simulink model "right_leg"  (R2014b)
settings: Solver=ode45  StartTime=0.0  StopTime=10  FixedStep=1e-3  RelTol=1e-3
undefined symbols (not defined in the file or in its folder): MX28_inertia, MX28_init_position, MX28_init_speed, MX28_Te, X, Y, Z
libraries: sm_lib x39, nesl_utility x20
(part 1 of 2)
settings Model: Creator=florent  LastModifiedBy=florent
settings DebuggingCC: IntegerOverflowMsg=none  ParameterDowncastMsg=warning  ParameterPrecisionLossMsg=none  ParameterTunabilityLossMsg=none  StateNameClashWarn=warning  IntegerSaturationMsg=none
settings DiagnosticsConfigSet: SimMechanicsConflictingReferenceFrames=none

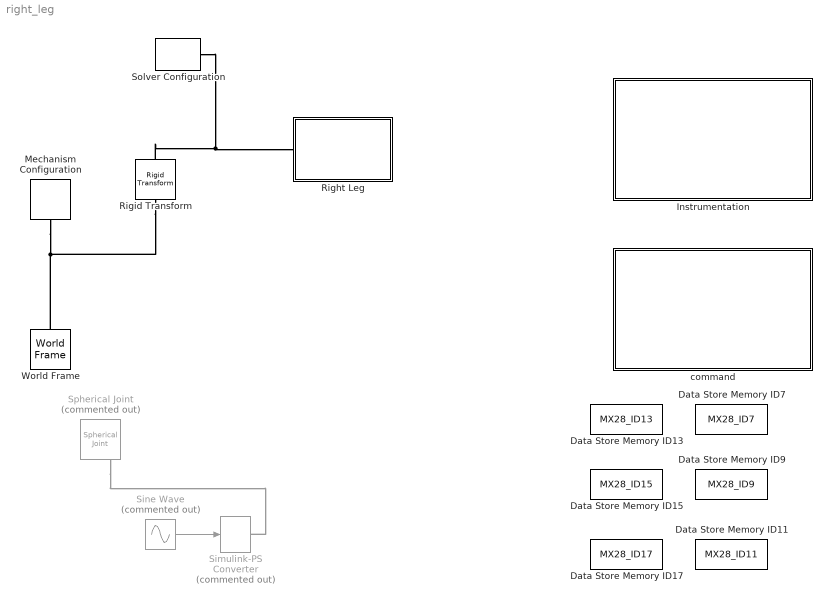
== system right_leg ==
  Data Store Memory ID11 : DataStoreMemory  DataStoreName=MX28_ID11  WriteAfterWriteMsg=error  InitialValue=MX28_default  VectorParams1D=off  OutDataTypeStr=Bus: MX28_bus
  Data Store Memory ID13 : DataStoreMemory  DataStoreName=MX28_ID13  WriteAfterWriteMsg=error  InitialValue=MX28_default  VectorParams1D=off  OutDataTypeStr=Bus: MX28_bus
  Data Store Memory ID15 : DataStoreMemory  DataStoreName=MX28_ID15  WriteAfterWriteMsg=error  InitialValue=MX28_default  VectorParams1D=off  OutDataTypeStr=Bus: MX28_bus
  Data Store Memory ID17 : DataStoreMemory  DataStoreName=MX28_ID17  WriteAfterWriteMsg=error  InitialValue=MX28_default  VectorParams1D=off  OutDataTypeStr=Bus: MX28_bus
  Data Store Memory ID7 : DataStoreMemory  DataStoreName=MX28_ID7  WriteAfterWriteMsg=error  InitialValue=MX28_default  VectorParams1D=off  OutDataTypeStr=Bus: MX28_bus
  Data Store Memory ID9 : DataStoreMemory  DataStoreName=MX28_ID9  WriteAfterWriteMsg=error  InitialValue=MX28_default  VectorParams1D=off  OutDataTypeStr=Bus: MX28_bus
  Instrumentation : Subsystem
  Mechanism Configuration : sm_lib/Utilities/Mechanism Configuration  UniformGravity=Constant  GravityVector=[0 0 -9.80665]  GravityUnits=m/s^2  LinearizationDelta=0.0001  BlockFunction=simmechanics.library.utilities.mechanism_configuration
  Right Leg : Subsystem
      mask init:
      | [ModelDir,~,~] = fileparts(which(gcs));
      | 
      | Block = [gcb '/Right Hip Yaw/Solid'];
      | STLFileName = [ModelDir filesep 'STL' filesep 'Hip1.STL'];
      | if ~strcmp(get_param(Block,'ExtGeomFileName'),STLFileName)
      |     set_param(Block,'ExtGeomFileName',STLFileName);
      | end
      | 
      | Block = [gcb '/Right Hip Roll/Solid'];
      | STLFileName = [ModelDir filesep 'STL' filesep 'Right_Hip2.STL'];
      | if ~strcmp(get_param(Block,'ExtGeomFileName'),STLFileName)
      |     set_param(Block,'ExtGeomFileName',STLFileName);
      | end
      | 
      | Block = [gcb '/Right Thigh/Solid'];
      | STLFileName = [ModelDir filesep 'STL' filesep 'Right_Thigh.STL'];
      | if ~strcmp(get_param(Block,'ExtGeomFileName'),STLFileName)
      |     set_param(Block,'ExtGeomFileName',STLFileName);
      | end
      | 
      | Block = [gcb '/Right Lower Leg/Solid'];
      | STLFileName = [ModelDir filesep 'STL' filesep 'Right_Lower_Leg.STL'];
      | if ~strcmp(get_param(Block,'ExtGeomFileName'),STLFileName)
      |     set_param(Block,'ExtGeomFileName',STLFileName);
      | end
      | 
      | Block = [gcb '/Right Ankle/Solid'];
      | STLFileName = [ModelDir filesep 'STL' filesep 'Right_Ankle.STL'];
      | if ~strcmp(get_param(Block,'ExtGeomFileName'),STLFileName)
      |     set_param(Block,'ExtGeomFileName',STLFileName);
      | end
      | 
      | Block = [gcb '/Right Foot/Solid'];
      | STLFileName = [ModelDir filesep 'STL' filesep 'Right_Foot.STL'];
      | if ~strcmp(get_param(Block,'ExtGeomFileName'),STLFileName)
      |     set_param(Block,'ExtGeomFileName',STLFileName);
      | end
  Rigid Transform : sm_lib/Frames and Transforms/Rigid Transform  TranslationMethod=Cartesian  TranslationLengthUnit=m  TranslationStandardAxis=+Z  TranslationStandardOffset=0  TranslationCartesianOffset=[0 -0.001 0]  TranslationROffset=0  TranslationROffsetUnits=m  TranslationZOffset=0  TranslationZOffsetUnits=m  TranslationThetaOffset=0  TranslationThetaOffsetUnits=deg  RotationMethod=AlignedAxes  RotationAngleUnits=deg  RotationStandardAxis=+Z  RotationAngle=0  RotationArbitraryAxis=[0 0 1]  FollAlignAxisA=+Z  BaseAlignAxisA=-Z  FollAlignAxisB=+X  BaseAlignAxisB=-Y  RotationMatrix=[1 0 0; 0 1 0; 0 0 1]  BlockFunction=simmechanics.library.frames_transforms.rigid_transform
  Simulink-PS Converter : nesl_utility/Simulink-PS Converter  Commented=on  PhysicalDomain=network_engine_domain  SubClassName=ps_input  LeftPortType=input  RightPortType=output  PseudoPeriodic=off  Frequencies=[]  NoiseDistribution=none  NoiseParameters=[]  Unit=1  AffineConversion=off  InputFiltering=off  SimscapeFilterOrder=1  InputFilterTimeConstant=0.001  UdotUserProvided=1
  Sine Wave : Sin  Commented=on  Amplitude=0.1  Frequency=10  SampleTime=0
  Solver Configuration : nesl_utility/Solver Configuration  PhysicalDomain=network_engine_domain  SubClassName=solver  LeftPortType=input  RightPortType=generic  Accelerate=off  Tones=[]  Harmonics=[]  SimulateNoise=off  Profile=off  UseLocalSampling=off  EnableSwitchedLinearOptims=on  FrequencyDomain=off  UseCCode=off  RelTol=0.001  AbsTol=1e-06  MinStep=1e-09  ToWorkspace=off  DoDC=off  ResidualTolerance=1e-05  UseLocalSolver=off  LocalSolverChoice=NE_BACKWARD_EULER_ADVANCER  LocalSolverSampleTime=0.001  DoFixedCost=off  MaxNonlinIter=3  MaxModeIter=2  LinearAlgebra=Sparse  DelaysMemoryBudget=1024  AutomaticFiltering=on  FilteringTimeConstant=0.001
  Spherical Joint : sm_lib/Joints/Spherical Joint  Commented=on  SenseConstraintForce=off  SenseConstraintForceX=off  SenseConstraintForceY=off  SenseConstraintForceZ=off  SenseConstraintTorque=off  SenseConstraintTorqueX=off  SenseConstraintTorqueY=off  SenseConstraintTorqueZ=off  SenseTotalForce=off  SenseTotalForceX=off  SenseTotalForceY=off  SenseTotalForceZ=off  SenseTotalTorque=off  SenseTotalTorqueX=off  SenseTotalTorqueY=off  SenseTotalTorqueZ=off  CompositeWrenchDir=FollowerOnBase  CompositeWrenchFrame=BaseFrame  DefPosRotationMethod=None  DefPosRotationAngleUnits=deg  DefPosRotationStandardAxis=+Z  DefPosRotationAngle=0  DefPosRotationArbitraryAxis=[0 0 1]  DefPosFollAlignAxisA=+X  DefPosBaseAlignAxisA=+Y  DefPosFollAlignAxisB=+Y  DefPosBaseAlignAxisB=+Z  DefPosRotationMatrix=[1 0 0; 0 1 0; 0 0 1]  EqPosRotationMethod=None  EqPosRotationAngleUnits=deg  EqPosRotationStandardAxis=+Z  EqPosRotationAngle=0  EqPosRotationArbitraryAxis=[0 0 1]  EqPosFollAlignAxisA=+X  EqPosBaseAlignAxisA=+Y  EqPosFollAlignAxisB=+Y  EqPosBaseAlignAxisB=+Z  EqPosRotationMatrix=[1 0 0; 0 1 0; 0 0 1]  SpringStiffness=0  SpringStiffnessUnits=N*m/deg  DampingCoefficient=0  DampingCoefficientUnits=N*m/(deg/s)  ActuateTorqueX=off  ActuateTorqueY=on  ActuateTorqueZ=off  ActuateTorque=off  TorqueActuationMode=InputTorque  MotionActuationMode=ComputedMotion  ActuationFrame=BaseFrame  SensePosition=off  SenseVelocityX=off  SenseVelocityY=off  SenseVelocityZ=off  SenseVelocity=off  SenseAccelerationX=off  SenseAccelerationY=off  SenseAccelerationZ=off  SenseAcceleration=off  SenseTorqueX=off  SenseTorqueY=off  SenseTorqueZ=off  SenseTorqueForce=off  SensingFrame=BaseFrame  PositionTargetRotationMethod=ArbitraryAxis  PositionTargetRotationAngleUnits=deg  PositionTargetRotationStandardAxis=+Z  PositionTargetRotationAngle=0  PositionTargetRotationArbitraryAxis=[0 -1 0]  PositionTargetFollAlignAxisA=+X  PositionTargetBaseAlignAxisA=+Y  PositionTargetFollAlignAxisB=+Y  PositionTargetBaseAlignAxisB=+Z  PositionTargetRotationMatrix=[1 0 0; 0 1 0; 0 0 1]  PositionTargetSpecify=on  PositionTargetPriority=High  VelocityTargetValue=[0 0 0]  VelocityTargetValueUnits=deg/s  VelocityTargetSpecify=off  VelocityTargetPriority=High  VelocityTargetInFollowerFrame=on  BlockFunction=simmechanics.library.joints.spherical_joint
  World Frame : sm_lib/Frames and Transforms/World Frame  BlockFunction=simmechanics.library.frames_transforms.world_frame
  command : Subsystem
  wires:
  Sine Wave/1 -> Simulink-PS Converter/1
  connections:
  Solver Configuration/RConn1 -- Rigid Transform/RConn1 -- Right Leg/LConn1
  World Frame/RConn1 -- Rigid Transform/LConn1 -- Mechanism Configuration/RConn1
  Spherical Joint/LConn2 -- Simulink-PS Converter/RConn1

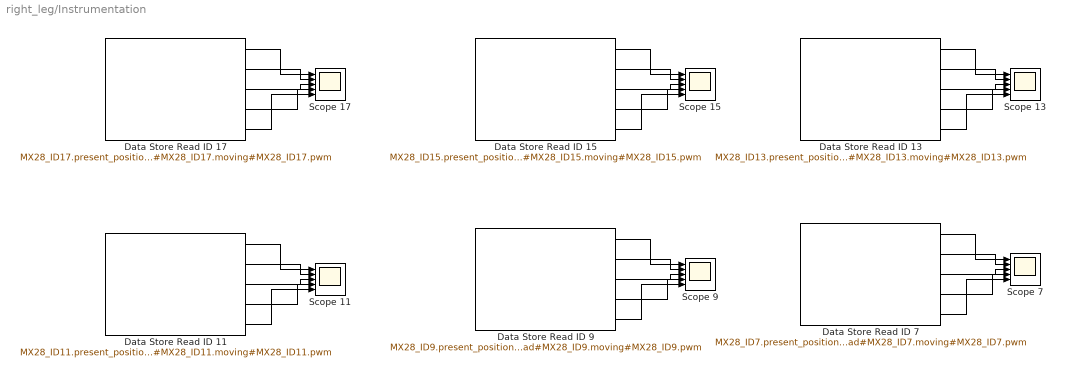
== system right_leg/Instrumentation ==
  Data Store Read ID 11 : DataStoreRead  DataStoreName=MX28_ID11  SampleTime=0.001  DataStoreElements=MX28_ID11.present_position#MX28_ID11.present_speed#MX28_ID11.present_load#MX28_ID11.moving#MX28_ID11.pwm
  Data Store Read ID 13 : DataStoreRead  DataStoreName=MX28_ID13  SampleTime=0.001  DataStoreElements=MX28_ID13.present_position#MX28_ID13.present_speed#MX28_ID13.present_load#MX28_ID13.moving#MX28_ID13.pwm
  Data Store Read ID 15 : DataStoreRead  DataStoreName=MX28_ID15  SampleTime=0.001  DataStoreElements=MX28_ID15.present_position#MX28_ID15.present_speed#MX28_ID15.present_load#MX28_ID15.moving#MX28_ID15.pwm
  Data Store Read ID 17 : DataStoreRead  DataStoreName=MX28_ID17  SampleTime=0.001  DataStoreElements=MX28_ID17.present_position#MX28_ID17.present_speed#MX28_ID17.present_load#MX28_ID17.moving#MX28_ID17.pwm
  Data Store Read ID 7 : DataStoreRead  DataStoreName=MX28_ID7  SampleTime=0.001  DataStoreElements=MX28_ID7.present_position#MX28_ID7.present_speed#MX28_ID7.present_load#MX28_ID7.moving#MX28_ID7.pwm
  Data Store Read ID 9 : DataStoreRead  DataStoreName=MX28_ID9  SampleTime=0.001  DataStoreElements=MX28_ID9.present_position#MX28_ID9.present_speed#MX28_ID9.present_load#MX28_ID9.moving#MX28_ID9.pwm
  Scope {7,9,11,13,15,17} (6 alike) : Scope  NumInputPorts=5
      Scope 11 settings: YMin=-5~0~-5~-5~-5  YMax=5~650~5~5~5
      Scope 13 settings: YMin=2046~-5~-40~-1~0  YMax=2047~5~0~1~20
      Scope 15 settings: YMin=2049~-5~0~-1~-20  YMax=2050~5~40~1~0  SaveName=ScopeData3
      Scope 17 settings: YMin=2048~-5~-20~-1~-10  YMax=2049~5~20~1~0  SaveName=ScopeData4
      Scope 7 settings: YMin=-5~0~-5~-5~-5  YMax=5~650~5~5~5  SaveName=ScopeData6
      Scope 9 settings: YMin=-5~0~-5~-5~-5  YMax=5~650~5~5~5  SaveName=ScopeData5
  wires:
  Data Store Read ID 13/1 -> Scope 13/1
  Data Store Read ID 13/2 -> Scope 13/2
  Data Store Read ID 13/3 -> Scope 13/3
  Data Store Read ID 13/4 -> Scope 13/4
  Data Store Read ID 13/5 -> Scope 13/5
  Data Store Read ID 15/1 -> Scope 15/1
  Data Store Read ID 15/2 -> Scope 15/2
  Data Store Read ID 15/3 -> Scope 15/3
  Data Store Read ID 15/4 -> Scope 15/4
  Data Store Read ID 15/5 -> Scope 15/5
  Data Store Read ID 17/1 -> Scope 17/1
  Data Store Read ID 17/2 -> Scope 17/2
  Data Store Read ID 17/3 -> Scope 17/3
  Data Store Read ID 17/4 -> Scope 17/4
  Data Store Read ID 17/5 -> Scope 17/5
  Data Store Read ID 11/1 -> Scope 11/1
  Data Store Read ID 11/2 -> Scope 11/2
  Data Store Read ID 11/3 -> Scope 11/3
  Data Store Read ID 11/4 -> Scope 11/4
  Data Store Read ID 11/5 -> Scope 11/5
  Data Store Read ID 9/1 -> Scope 9/1
  Data Store Read ID 9/2 -> Scope 9/2
  Data Store Read ID 9/3 -> Scope 9/3
  Data Store Read ID 9/4 -> Scope 9/4
  Data Store Read ID 9/5 -> Scope 9/5
  Data Store Read ID 7/1 -> Scope 7/1
  Data Store Read ID 7/2 -> Scope 7/2
  Data Store Read ID 7/3 -> Scope 7/3
  Data Store Read ID 7/4 -> Scope 7/4
  Data Store Read ID 7/5 -> Scope 7/5

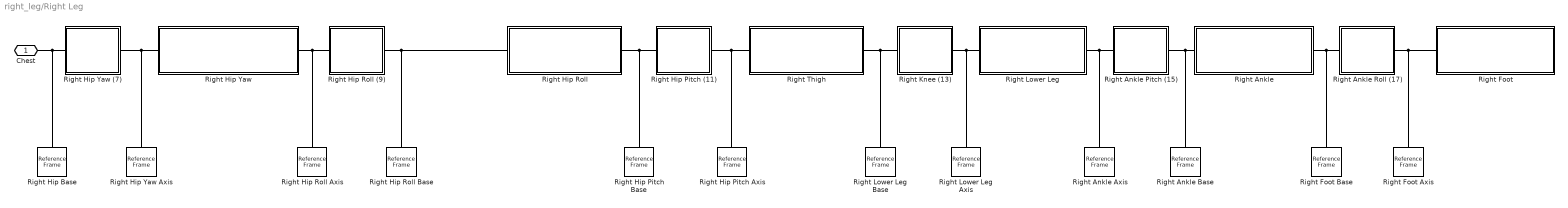
== system right_leg/Right Leg ==
  Right Ankle : Subsystem
  Right Ankle Axis : sm_lib/Frames and Transforms/Reference Frame  BlockFunction=simmechanics.library.frames_transforms.reference_frame
  Right Ankle Base : sm_lib/Frames and Transforms/Reference Frame  BlockFunction=simmechanics.library.frames_transforms.reference_frame
  Right Ankle Pitch (15) : Subsystem
  Right Ankle Roll (17) : Subsystem
  Right Foot : Subsystem
  Right Foot Axis : sm_lib/Frames and Transforms/Reference Frame  BlockFunction=simmechanics.library.frames_transforms.reference_frame
  Right Foot Base : sm_lib/Frames and Transforms/Reference Frame  BlockFunction=simmechanics.library.frames_transforms.reference_frame
  Right Hip Base : sm_lib/Frames and Transforms/Reference Frame  BlockFunction=simmechanics.library.frames_transforms.reference_frame
  Right Hip Pitch (11) : Subsystem
  Right Hip Pitch Axis : sm_lib/Frames and Transforms/Reference Frame  BlockFunction=simmechanics.library.frames_transforms.reference_frame
  Right Hip Pitch Base : sm_lib/Frames and Transforms/Reference Frame  BlockFunction=simmechanics.library.frames_transforms.reference_frame
  Right Hip Roll : Subsystem
  Right Hip Roll (9) : Subsystem
  Right Hip Roll Axis : sm_lib/Frames and Transforms/Reference Frame  BlockFunction=simmechanics.library.frames_transforms.reference_frame
  Right Hip Roll Base : sm_lib/Frames and Transforms/Reference Frame  BlockFunction=simmechanics.library.frames_transforms.reference_frame
  Right Hip Yaw : Subsystem
  Right Hip Yaw (7) : Subsystem
  Right Hip Yaw Axis : sm_lib/Frames and Transforms/Reference Frame  BlockFunction=simmechanics.library.frames_transforms.reference_frame
  Right Knee (13) : Subsystem
  Right Lower Leg : Subsystem
  Right Lower Leg Axis : sm_lib/Frames and Transforms/Reference Frame  BlockFunction=simmechanics.library.frames_transforms.reference_frame
  Right Lower Leg Base : sm_lib/Frames and Transforms/Reference Frame  BlockFunction=simmechanics.library.frames_transforms.reference_frame
  Right Thigh : Subsystem
  Chest : PMIOPort  Port=1  Side=Left
  connections:
  Chest/RConn1 -- Right Hip Yaw (7)/LConn1 -- Right Hip Base/RConn1
  Right Hip Yaw Axis/RConn1 -- Right Hip Yaw (7)/RConn1 -- Right Hip Yaw/LConn1
  Right Hip Yaw/RConn1 -- Right Hip Roll (9)/RConn1 -- Right Hip Roll Axis/RConn1
  Right Hip Roll/RConn1 -- Right Hip Pitch Base/RConn1 -- Right Hip Pitch (11)/LConn1
  Right Thigh/RConn1 -- Right Lower Leg Base/RConn1 -- Right Knee (13)/LConn1
  Right Ankle/RConn1 -- Right Foot Base/RConn1 -- Right Ankle Roll (17)/LConn1
  Right Thigh/LConn1 -- Right Hip Pitch (11)/RConn1 -- Right Hip Pitch Axis/RConn1
  Right Lower Leg/LConn1 -- Right Knee (13)/RConn1 -- Right Lower Leg Axis/RConn1
  Right Lower Leg/RConn1 -- Right Ankle Axis/RConn1 -- Right Ankle Pitch (15)/RConn1
  Right Ankle/LConn1 -- Right Ankle Pitch (15)/LConn1 -- Right Ankle Base/RConn1
  Right Ankle Roll (17)/RConn1 -- Right Foot/LConn1 -- Right Foot Axis/RConn1
  Right Hip Roll Base/RConn1 -- Right Hip Roll (9)/LConn1 -- Right Hip Roll/LConn1

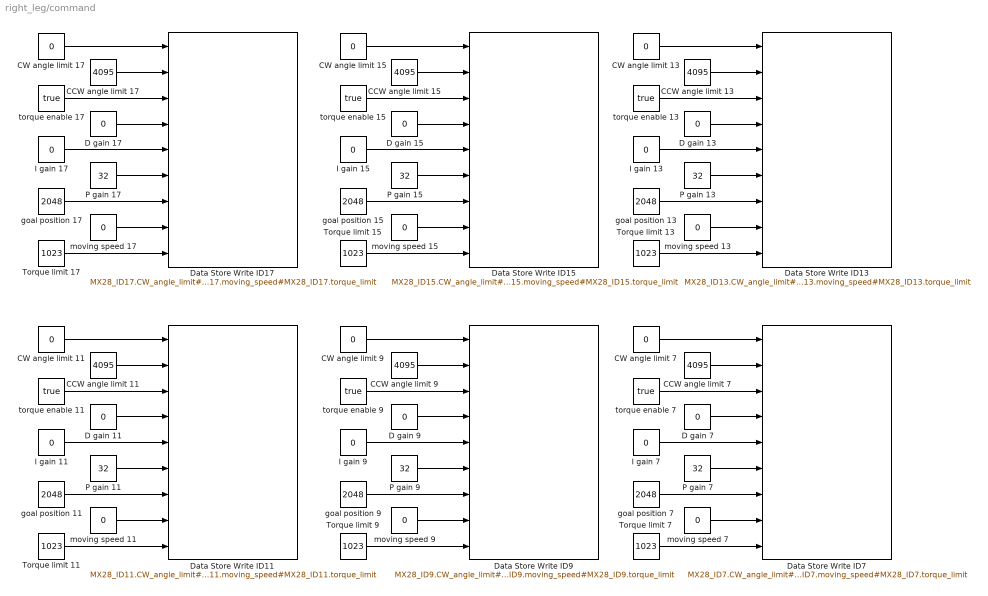
== system right_leg/command ==
  CCW angle limit {7,9,11,13,15,17} (6 alike) : Constant  Value=4095  OutDataTypeStr=int16
  CW angle limit {7,9,11,13,15,17} (6 alike) : Constant  Value=0  OutDataTypeStr=int16
  D gain {7,9,11,13,15,17} (6 alike) : Constant  Value=0  OutDataTypeStr=uint8
  Data Store Write ID11 : DataStoreWrite  DataStoreName=MX28_ID11  DataStoreElements=MX28_ID11.CW_angle_limit#MX28_ID11.CCW_angle_limit#MX28_ID11.torque_enable#MX28_ID11.D_gain#MX28_ID11.I_gain#MX28_ID11.P_gain#MX28_ID11.goal_position#MX28_ID11.moving_speed#MX28_ID11.torque_limit
  Data Store Write ID13 : DataStoreWrite  DataStoreName=MX28_ID13  DataStoreElements=MX28_ID13.CW_angle_limit#MX28_ID13.CCW_angle_limit#MX28_ID13.torque_enable#MX28_ID13.D_gain#MX28_ID13.I_gain#MX28_ID13.P_gain#MX28_ID13.goal_position#MX28_ID13.moving_speed#MX28_ID13.torque_limit
  Data Store Write ID15 : DataStoreWrite  DataStoreName=MX28_ID15  DataStoreElements=MX28_ID15.CW_angle_limit#MX28_ID15.CCW_angle_limit#MX28_ID15.torque_enable#MX28_ID15.D_gain#MX28_ID15.I_gain#MX28_ID15.P_gain#MX28_ID15.goal_position#MX28_ID15.moving_speed#MX28_ID15.torque_limit
  Data Store Write ID17 : DataStoreWrite  DataStoreName=MX28_ID17  DataStoreElements=MX28_ID17.CW_angle_limit#MX28_ID17.CCW_angle_limit#MX28_ID17.torque_enable#MX28_ID17.D_gain#MX28_ID17.I_gain#MX28_ID17.P_gain#MX28_ID17.goal_position#MX28_ID17.moving_speed#MX28_ID17.torque_limit
  Data Store Write ID7 : DataStoreWrite  DataStoreName=MX28_ID7  DataStoreElements=MX28_ID7.CW_angle_limit#MX28_ID7.CCW_angle_limit#MX28_ID7.torque_enable#MX28_ID7.D_gain#MX28_ID7.I_gain#MX28_ID7.P_gain#MX28_ID7.goal_position#MX28_ID7.moving_speed#MX28_ID7.torque_limit
  Data Store Write ID9 : DataStoreWrite  DataStoreName=MX28_ID9  DataStoreElements=MX28_ID9.CW_angle_limit#MX28_ID9.CCW_angle_limit#MX28_ID9.torque_enable#MX28_ID9.D_gain#MX28_ID9.I_gain#MX28_ID9.P_gain#MX28_ID9.goal_position#MX28_ID9.moving_speed#MX28_ID9.torque_limit
  I gain {7,9,11,13,15,17} (6 alike) : Constant  Value=0  OutDataTypeStr=uint8
  P gain {7,9,11,13,15,17} (6 alike) : Constant  Value=32  OutDataTypeStr=uint8
  Torque limit {7,9,11,13,15,17} (6 alike) : Constant  Value=1023  OutDataTypeStr=int16
  goal position {7,9,11,13,15,17} (6 alike) : Constant  Value=2048  OutDataTypeStr=int16
  moving speed {7,9,11,13,15,17} (6 alike) : Constant  Value=0  OutDataTypeStr=int16
  torque enable {7,9,11,13,15,17} (6 alike) : Constant  Value=true  OutDataTypeStr=boolean
  wires:
  Torque limit 17/1 -> Data Store Write ID17/9
  moving speed 17/1 -> Data Store Write ID17/8
  goal position 17/1 -> Data Store Write ID17/7
  P gain 17/1 -> Data Store Write ID17/6
  I gain 17/1 -> Data Store Write ID17/5
  D gain 17/1 -> Data Store Write ID17/4
  torque enable 17/1 -> Data Store Write ID17/3
  CW angle limit 17/1 -> Data Store Write ID17/1
  CCW angle limit 17/1 -> Data Store Write ID17/2
  Torque limit 15/1 -> Data Store Write ID15/9
  moving speed 15/1 -> Data Store Write ID15/8
  goal position 15/1 -> Data Store Write ID15/7
  P gain 15/1 -> Data Store Write ID15/6
  I gain 15/1 -> Data Store Write ID15/5
  D gain 15/1 -> Data Store Write ID15/4
  torque enable 15/1 -> Data Store Write ID15/3
  CCW angle limit 15/1 -> Data Store Write ID15/2
  CW angle limit 15/1 -> Data Store Write ID15/1
  Torque limit 13/1 -> Data Store Write ID13/9
  moving speed 13/1 -> Data Store Write ID13/8
  goal position 13/1 -> Data Store Write ID13/7
  P gain 13/1 -> Data Store Write ID13/6
  I gain 13/1 -> Data Store Write ID13/5
  D gain 13/1 -> Data Store Write ID13/4
  torque enable 13/1 -> Data Store Write ID13/3
  CW angle limit 13/1 -> Data Store Write ID13/1
  CCW angle limit 13/1 -> Data Store Write ID13/2
  Torque limit 11/1 -> Data Store Write ID11/9
  moving speed 11/1 -> Data Store Write ID11/8
  goal position 11/1 -> Data Store Write ID11/7
  P gain 11/1 -> Data Store Write ID11/6
  I gain 11/1 -> Data Store Write ID11/5
  D gain 11/1 -> Data Store Write ID11/4
  torque enable 11/1 -> Data Store Write ID11/3
  CW angle limit 11/1 -> Data Store Write ID11/1
  CCW angle limit 11/1 -> Data Store Write ID11/2
  Torque limit 9/1 -> Data Store Write ID9/9
  moving speed 9/1 -> Data Store Write ID9/8
  goal position 9/1 -> Data Store Write ID9/7
  P gain 9/1 -> Data Store Write ID9/6
  I gain 9/1 -> Data Store Write ID9/5
  D gain 9/1 -> Data Store Write ID9/4
  torque enable 9/1 -> Data Store Write ID9/3
  CW angle limit 9/1 -> Data Store Write ID9/1
  CCW angle limit 9/1 -> Data Store Write ID9/2
  Torque limit 7/1 -> Data Store Write ID7/9
  moving speed 7/1 -> Data Store Write ID7/8
  goal position 7/1 -> Data Store Write ID7/7
  P gain 7/1 -> Data Store Write ID7/6
  I gain 7/1 -> Data Store Write ID7/5
  D gain 7/1 -> Data Store Write ID7/4
  torque enable 7/1 -> Data Store Write ID7/3
  CW angle limit 7/1 -> Data Store Write ID7/1
  CCW angle limit 7/1 -> Data Store Write ID7/2

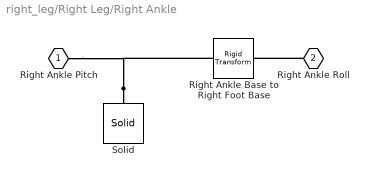
== system right_leg/Right Leg/Right Ankle ==
  Right Ankle Base to Right Foot Base : sm_lib/Frames and Transforms/Rigid Transform  TranslationMethod=Cartesian  TranslationLengthUnit=mm  TranslationStandardAxis=+Z  TranslationStandardOffset=0  TranslationCartesianOffset=[-19.35 0 -24]  TranslationROffset=0  TranslationROffsetUnits=m  TranslationZOffset=0  TranslationZOffsetUnits=m  TranslationThetaOffset=0  TranslationThetaOffsetUnits=deg  RotationMethod=AlignedAxes  RotationAngleUnits=deg  RotationStandardAxis=+Z  RotationAngle=0  RotationArbitraryAxis=[0 0 1]  FollAlignAxisA=+X  BaseAlignAxisA=+Z  FollAlignAxisB=+Y  BaseAlignAxisB=-Y  RotationMatrix=[1 0 0; 0 1 0; 0 0 1]  BlockFunction=simmechanics.library.frames_transforms.rigid_transform
  Solid : sm_lib/Body Elements/Solid  InertiaType=Custom  Mass=166.79  MassUnits=g  CenterOfMass=[-18.06 -11.21 -24.20]  CenterOfMassUnits=mm  MomentsOfInertia=[6948 12212 11817]  MomentsOfInertiaUnits=g*mm^2  ProductsOfInertia=[-194 117 4006]  ProductsOfInertiaUnits=g*mm^2  DensityBased=on  Density=1000  DensityUnits=kg/(m^3)  GraphicType=FromGeometry  MarkerShape=Sphere  MarkerSize=10  MarkerSizeUnits=m  GraphicVisPropType=SimpleVisualProperties  GraphicDiffuseColor=[0.5 0.5 0.5]  GraphicSpecularColor=[0.5 0.5 0.5 1.0]  GraphicAmbientColor=[0.15 0.15 0.15 1.0]  GraphicEmissiveColor=[0.0 0.0 0.0 1.0]  GraphicShininess=75  GraphicOpacity=1.0  GeometryShape=FromFile  RectangleSize=[1 1]  RectangleSizeUnits=m  BrickDimensions=[1 1 1]  BrickDimensionUnits=m  CylinderRadius=1  CylinderRadiusUnits=m  CylinderLength=1  CylinderLengthUnits=m  SphereRadius=1  SphereRadiusUnits=m  EllipsoidRadii=[1 1 1]  EllipsoidRadiiUnits=m  ExtrusionCrossSection=[1 1; -1 1; -1 -1; 1 -1]  ExtrusionCrossSectionUnits=m  ExtrusionLength=1  ExtrusionLengthUnits=m  PolygonNumSides=3  PolygonOuterRadius=1  PolygonOuterRadiusUnits=m  ExtGeomFileType=STL  ExtGeomFileName=D:\Ker Lann\systemes\darwin\kinematics\STL\Right_Ankle.STL  ExtGeomFileUnits=mm  RevolutionCrossSection=[1 1; 1 -1; 2 -1; 2 1]  RevolutionCrossSectionUnits=m  RevolutionExtent=Full  RevolutionAngle=180  RevolutionAngleUnits=deg  BlockFunction=simmechanics.library.body_elements.solid
  Right Ankle Pitch : PMIOPort  Port=1  Side=Left
  Right Ankle Roll : PMIOPort  Port=2  Side=Right
  connections:
  Solid/RConn1 -- Right Ankle Base to Right Foot Base/LConn1 -- Right Ankle Pitch/RConn1
  Right Ankle Roll/RConn1 -- Right Ankle Base to Right Foot Base/RConn1

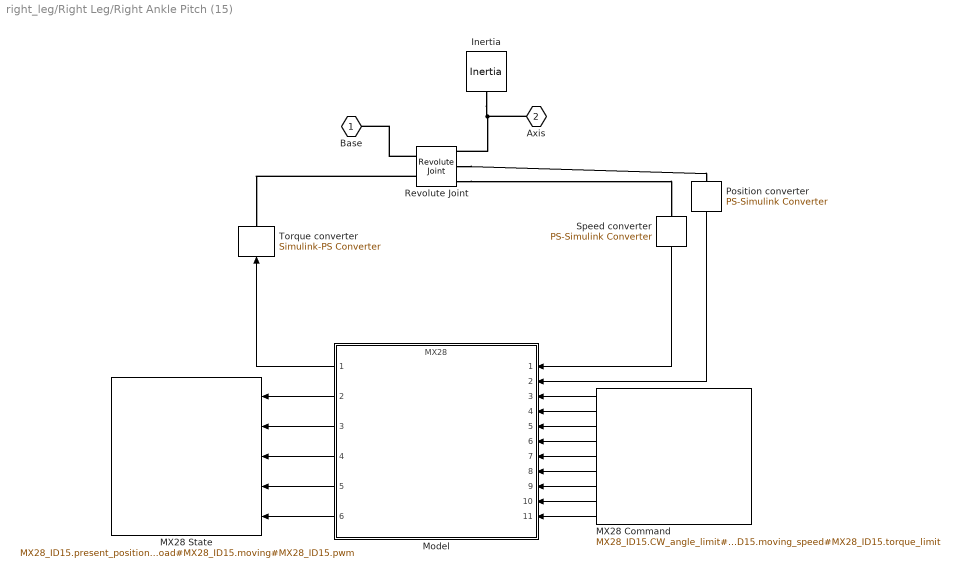
== system right_leg/Right Leg/Right Ankle Pitch (15) ==
  Inertia : sm_lib/Body Elements/Inertia  InertiaType=Custom  Mass=1  MassUnits=g  CenterOfMass=[0 0 0]  CenterOfMassUnits=m  MomentsOfInertia=[0 0 MX28_inertia]  MomentsOfInertiaUnits=kg*m^2  ProductsOfInertia=[0 0 0]  ProductsOfInertiaUnits=kg*m^2  BlockFunction=simmechanics.library.body_elements.inertia
  MX28 Command : DataStoreRead  DataStoreName=MX28_ID15  SampleTime=MX28_Te  DataStoreElements=MX28_ID15.CW_angle_limit#MX28_ID15.CCW_angle_limit#MX28_ID15.torque_enable#MX28_ID15.D_gain#MX28_ID15.I_gain#MX28_ID15.P_gain#MX28_ID15.goal_position#MX28_ID15.moving_speed#MX28_ID15.torque_limit
  MX28 State : DataStoreWrite  DataStoreName=MX28_ID15  DataStoreElements=MX28_ID15.present_position#MX28_ID15.present_speed#MX28_ID15.present_load#MX28_ID15.moving#MX28_ID15.pwm
  Model : ModelReference  ModelNameDialog=MX28.slx  SimulationMode=Normal  ModelReferenceVersion=1.66  CopyOfModelName=MX28.slx  DefaultDataLogging=on
  Position converter : nesl_utility/PS-Simulink Converter  PhysicalDomain=network_engine_domain  SubClassName=ps_output  LeftPortType=input  RightPortType=output  PseudoPeriodic=off  Frequencies=[]  Unit=rad  AffineConversion=off
  Revolute Joint : sm_lib/Joints/Revolute Joint  SenseConstraintForce=off  SenseConstraintForceX=off  SenseConstraintForceY=off  SenseConstraintForceZ=off  SenseConstraintTorque=off  SenseConstraintTorqueX=off  SenseConstraintTorqueY=off  SenseConstraintTorqueZ=off  SenseTotalForce=off  SenseTotalForceX=off  SenseTotalForceY=off  SenseTotalForceZ=off  SenseTotalTorque=off  SenseTotalTorqueX=off  SenseTotalTorqueY=off  SenseTotalTorqueZ=off  CompositeWrenchDir=FollowerOnBase  CompositeWrenchFrame=BaseFrame  EquilibriumPosition=0  EquilibriumPositionUnits=deg  SpringStiffness=0  SpringStiffnessUnits=N*m/deg  DampingCoefficient=MX28_lub_friction  DampingCoefficientUnits=N*m/(rad/s)  TorqueActuationMode=InputTorque  MotionActuationMode=ComputedMotion  SensePosition=on  SenseVelocity=on  SenseAcceleration=off  SenseTorqueForce=off  PositionTargetValue=MX28_init_position  PositionTargetValueUnits=rad  PositionTargetSpecify=on  PositionTargetPriority=High  VelocityTargetValue=MX28_init_speed  VelocityTargetValueUnits=rad/s  VelocityTargetSpecify=on  VelocityTargetPriority=High  BlockFunction=simmechanics.library.joints.revolute_joint
  Speed converter : nesl_utility/PS-Simulink Converter  PhysicalDomain=network_engine_domain  SubClassName=ps_output  LeftPortType=input  RightPortType=output  PseudoPeriodic=off  Frequencies=[]  Unit=rad/s  AffineConversion=off
  Torque converter : nesl_utility/Simulink-PS Converter  PhysicalDomain=network_engine_domain  SubClassName=ps_input  LeftPortType=input  RightPortType=output  PseudoPeriodic=off  Frequencies=[]  NoiseDistribution=none  NoiseParameters=[]  Unit=N*m  AffineConversion=off  InputFiltering=off  SimscapeFilterOrder=1  InputFilterTimeConstant=0.001  UdotUserProvided=1
  Base : PMIOPort  Port=1  Side=Left
  Axis : PMIOPort  Port=2  Side=Right
  wires:
  Model/4 -> MX28 State/3
  Model/2 -> MX28 State/1
  Model/5 -> MX28 State/4
  Model/3 -> MX28 State/2
  MX28 Command/3 -> Model/5
  MX28 Command/6 -> Model/8
  MX28 Command/4 -> Model/6
  MX28 Command/5 -> Model/7
  MX28 Command/7 -> Model/9
  MX28 Command/2 -> Model/4
  MX28 Command/1 -> Model/3
  Model/6 -> MX28 State/5
  MX28 Command/8 -> Model/10
  MX28 Command/9 -> Model/11
  Model/1 -> Torque converter/1
  Speed converter/1 -> Model/1
  Position converter/1 -> Model/2
  connections:
  Inertia/RConn1 -- Axis/RConn1 -- Revolute Joint/RConn1
  Revolute Joint/LConn1 -- Base/RConn1
  Revolute Joint/RConn3 -- Speed converter/LConn1
  Revolute Joint/RConn2 -- Position converter/LConn1
  Revolute Joint/LConn2 -- Torque converter/RConn1

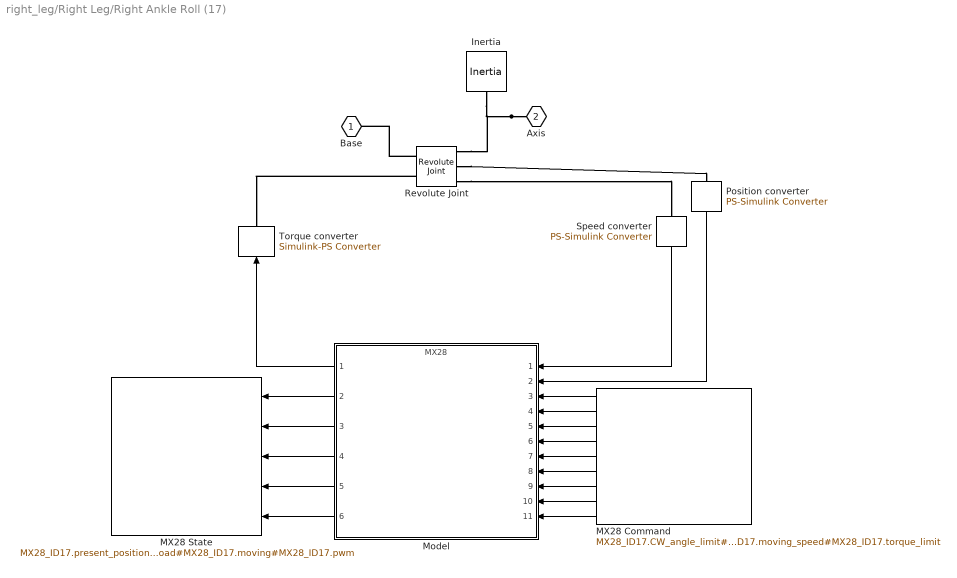
== system right_leg/Right Leg/Right Ankle Roll (17) ==
  Inertia : sm_lib/Body Elements/Inertia  InertiaType=Custom  Mass=1  MassUnits=g  CenterOfMass=[0 0 0]  CenterOfMassUnits=m  MomentsOfInertia=[0 0 MX28_inertia]  MomentsOfInertiaUnits=kg*m^2  ProductsOfInertia=[0 0 0]  ProductsOfInertiaUnits=kg*m^2  BlockFunction=simmechanics.library.body_elements.inertia
  MX28 Command : DataStoreRead  DataStoreName=MX28_ID17  SampleTime=MX28_Te  DataStoreElements=MX28_ID17.CW_angle_limit#MX28_ID17.CCW_angle_limit#MX28_ID17.torque_enable#MX28_ID17.D_gain#MX28_ID17.I_gain#MX28_ID17.P_gain#MX28_ID17.goal_position#MX28_ID17.moving_speed#MX28_ID17.torque_limit
  MX28 State : DataStoreWrite  DataStoreName=MX28_ID17  DataStoreElements=MX28_ID17.present_position#MX28_ID17.present_speed#MX28_ID17.present_load#MX28_ID17.moving#MX28_ID17.pwm
  Model : ModelReference  ModelNameDialog=MX28.slx  SimulationMode=Normal  ModelReferenceVersion=1.66  CopyOfModelName=MX28.slx  DefaultDataLogging=on
  Position converter : nesl_utility/PS-Simulink Converter  PhysicalDomain=network_engine_domain  SubClassName=ps_output  LeftPortType=input  RightPortType=output  PseudoPeriodic=off  Frequencies=[]  Unit=rad  AffineConversion=off
  Revolute Joint : sm_lib/Joints/Revolute Joint  SenseConstraintForce=off  SenseConstraintForceX=off  SenseConstraintForceY=off  SenseConstraintForceZ=off  SenseConstraintTorque=off  SenseConstraintTorqueX=off  SenseConstraintTorqueY=off  SenseConstraintTorqueZ=off  SenseTotalForce=off  SenseTotalForceX=off  SenseTotalForceY=off  SenseTotalForceZ=off  SenseTotalTorque=off  SenseTotalTorqueX=off  SenseTotalTorqueY=off  SenseTotalTorqueZ=off  CompositeWrenchDir=FollowerOnBase  CompositeWrenchFrame=BaseFrame  EquilibriumPosition=0  EquilibriumPositionUnits=deg  SpringStiffness=0  SpringStiffnessUnits=N*m/deg  DampingCoefficient=MX28_lub_friction  DampingCoefficientUnits=N*m/(rad/s)  TorqueActuationMode=InputTorque  MotionActuationMode=ComputedMotion  SensePosition=on  SenseVelocity=on  SenseAcceleration=off  SenseTorqueForce=off  PositionTargetValue=MX28_init_position  PositionTargetValueUnits=rad  PositionTargetSpecify=on  PositionTargetPriority=High  VelocityTargetValue=MX28_init_speed  VelocityTargetValueUnits=rad/s  VelocityTargetSpecify=on  VelocityTargetPriority=High  BlockFunction=simmechanics.library.joints.revolute_joint
  Speed converter : nesl_utility/PS-Simulink Converter  PhysicalDomain=network_engine_domain  SubClassName=ps_output  LeftPortType=input  RightPortType=output  PseudoPeriodic=off  Frequencies=[]  Unit=rad/s  AffineConversion=off
  Torque converter : nesl_utility/Simulink-PS Converter  PhysicalDomain=network_engine_domain  SubClassName=ps_input  LeftPortType=input  RightPortType=output  PseudoPeriodic=off  Frequencies=[]  NoiseDistribution=none  NoiseParameters=[]  Unit=N*m  AffineConversion=off  InputFiltering=off  SimscapeFilterOrder=1  InputFilterTimeConstant=0.001  UdotUserProvided=1
  Base : PMIOPort  Port=1  Side=Left
  Axis : PMIOPort  Port=2  Side=Right
  wires:
  Model/4 -> MX28 State/3
  Model/2 -> MX28 State/1
  Model/5 -> MX28 State/4
  Model/3 -> MX28 State/2
  Model/1 -> Torque converter/1
  MX28 Command/3 -> Model/5
  MX28 Command/6 -> Model/8
  MX28 Command/4 -> Model/6
  MX28 Command/5 -> Model/7
  MX28 Command/7 -> Model/9
  MX28 Command/2 -> Model/4
  MX28 Command/1 -> Model/3
  Position converter/1 -> Model/2
  Speed converter/1 -> Model/1
  Model/6 -> MX28 State/5
  MX28 Command/8 -> Model/10
  MX28 Command/9 -> Model/11
  connections:
  Axis/RConn1 -- Revolute Joint/RConn1 -- Inertia/RConn1
  Revolute Joint/LConn1 -- Base/RConn1
  Revolute Joint/RConn3 -- Speed converter/LConn1
  Revolute Joint/RConn2 -- Position converter/LConn1
  Revolute Joint/LConn2 -- Torque converter/RConn1

== system right_leg/Right Leg/Right Foot ==
  Solid : sm_lib/Body Elements/Solid  InertiaType=Custom  Mass=76.78  MassUnits=g  CenterOfMass=[7.76 24.5 17.25]  CenterOfMassUnits=mm  MomentsOfInertia=[69069 85303 36676]  MomentsOfInertiaUnits=g*mm^2  ProductsOfInertia=[4062 778 2754]  ProductsOfInertiaUnits=g*mm^2  DensityBased=on  Density=1000  DensityUnits=kg/(m^3)  GraphicType=FromGeometry  MarkerShape=Sphere  MarkerSize=10  MarkerSizeUnits=m  GraphicVisPropType=SimpleVisualProperties  GraphicDiffuseColor=[0.5 0.5 0.5]  GraphicSpecularColor=[0.5 0.5 0.5 1.0]  GraphicAmbientColor=[0.15 0.15 0.15 1.0]  GraphicEmissiveColor=[0.0 0.0 0.0 1.0]  GraphicShininess=75  GraphicOpacity=1.0  GeometryShape=FromFile  RectangleSize=[1 1]  RectangleSizeUnits=m  BrickDimensions=[1 1 1]  BrickDimensionUnits=m  CylinderRadius=1  CylinderRadiusUnits=m  CylinderLength=1  CylinderLengthUnits=m  SphereRadius=1  SphereRadiusUnits=m  EllipsoidRadii=[1 1 1]  EllipsoidRadiiUnits=m  ExtrusionCrossSection=[1 1; -1 1; -1 -1; 1 -1]  ExtrusionCrossSectionUnits=m  ExtrusionLength=1  ExtrusionLengthUnits=m  PolygonNumSides=3  PolygonOuterRadius=1  PolygonOuterRadiusUnits=m  ExtGeomFileType=STL  ExtGeomFileName=D:\Ker Lann\systemes\darwin\kinematics\STL\Right_Foot.STL  ExtGeomFileUnits=mm  RevolutionCrossSection=[1 1; 1 -1; 2 -1; 2 1]  RevolutionCrossSectionUnits=m  RevolutionExtent=Full  RevolutionAngle=180  RevolutionAngleUnits=deg  BlockFunction=simmechanics.library.body_elements.solid
  Right Ankle Roll : PMIOPort  Port=1  Side=Left
  connections:
  Right Ankle Roll/RConn1 -- Solid/RConn1

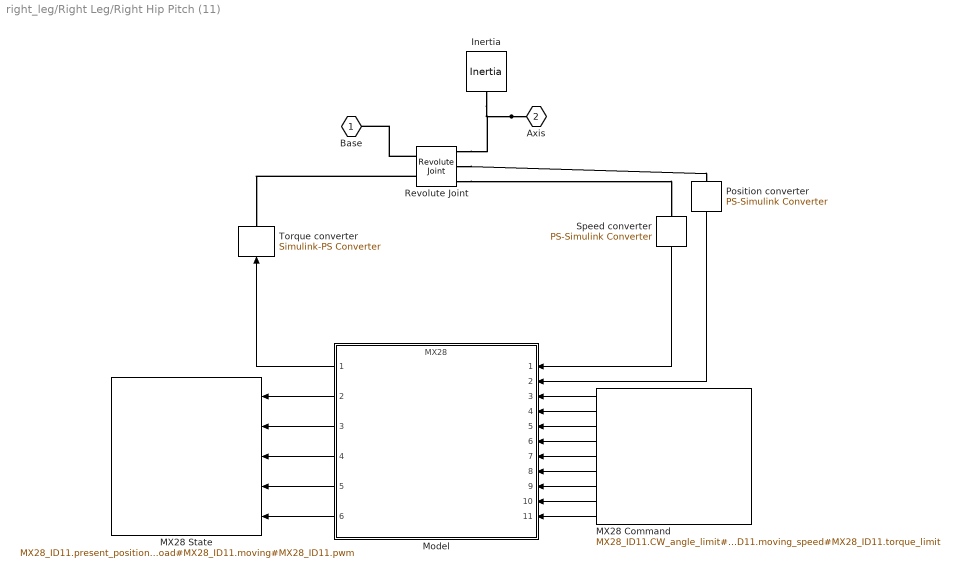
== system right_leg/Right Leg/Right Hip Pitch (11) ==
  Inertia : sm_lib/Body Elements/Inertia  InertiaType=Custom  Mass=1  MassUnits=g  CenterOfMass=[0 0 0]  CenterOfMassUnits=m  MomentsOfInertia=[0 0 MX28_inertia]  MomentsOfInertiaUnits=kg*m^2  ProductsOfInertia=[0 0 0]  ProductsOfInertiaUnits=kg*m^2  BlockFunction=simmechanics.library.body_elements.inertia
  MX28 Command : DataStoreRead  DataStoreName=MX28_ID11  SampleTime=MX28_Te  DataStoreElements=MX28_ID11.CW_angle_limit#MX28_ID11.CCW_angle_limit#MX28_ID11.torque_enable#MX28_ID11.D_gain#MX28_ID11.I_gain#MX28_ID11.P_gain#MX28_ID11.goal_position#MX28_ID11.moving_speed#MX28_ID11.torque_limit
  MX28 State : DataStoreWrite  DataStoreName=MX28_ID11  DataStoreElements=MX28_ID11.present_position#MX28_ID11.present_speed#MX28_ID11.present_load#MX28_ID11.moving#MX28_ID11.pwm
  Model : ModelReference  ModelNameDialog=MX28.slx  SimulationMode=Normal  ModelReferenceVersion=1.66  CopyOfModelName=MX28.slx  DefaultDataLogging=on
  Position converter : nesl_utility/PS-Simulink Converter  PhysicalDomain=network_engine_domain  SubClassName=ps_output  LeftPortType=input  RightPortType=output  PseudoPeriodic=off  Frequencies=[]  Unit=rad  AffineConversion=off
  Revolute Joint : sm_lib/Joints/Revolute Joint  SenseConstraintForce=off  SenseConstraintForceX=off  SenseConstraintForceY=off  SenseConstraintForceZ=off  SenseConstraintTorque=off  SenseConstraintTorqueX=off  SenseConstraintTorqueY=off  SenseConstraintTorqueZ=off  SenseTotalForce=off  SenseTotalForceX=off  SenseTotalForceY=off  SenseTotalForceZ=off  SenseTotalTorque=off  SenseTotalTorqueX=off  SenseTotalTorqueY=off  SenseTotalTorqueZ=off  CompositeWrenchDir=FollowerOnBase  CompositeWrenchFrame=BaseFrame  EquilibriumPosition=0  EquilibriumPositionUnits=deg  SpringStiffness=0  SpringStiffnessUnits=N*m/deg  DampingCoefficient=MX28_lub_friction  DampingCoefficientUnits=N*m/(rad/s)  TorqueActuationMode=InputTorque  MotionActuationMode=ComputedMotion  SensePosition=on  SenseVelocity=on  SenseAcceleration=off  SenseTorqueForce=off  PositionTargetValue=MX28_init_position  PositionTargetValueUnits=rad  PositionTargetSpecify=on  PositionTargetPriority=High  VelocityTargetValue=MX28_init_speed  VelocityTargetValueUnits=rad/s  VelocityTargetSpecify=on  VelocityTargetPriority=High  BlockFunction=simmechanics.library.joints.revolute_joint
  Speed converter : nesl_utility/PS-Simulink Converter  PhysicalDomain=network_engine_domain  SubClassName=ps_output  LeftPortType=input  RightPortType=output  PseudoPeriodic=off  Frequencies=[]  Unit=rad/s  AffineConversion=off
  Torque converter : nesl_utility/Simulink-PS Converter  PhysicalDomain=network_engine_domain  SubClassName=ps_input  LeftPortType=input  RightPortType=output  PseudoPeriodic=off  Frequencies=[]  NoiseDistribution=none  NoiseParameters=[]  Unit=N*m  AffineConversion=off  InputFiltering=off  SimscapeFilterOrder=1  InputFilterTimeConstant=0.001  UdotUserProvided=1
  Base : PMIOPort  Port=1  Side=Left
  Axis : PMIOPort  Port=2  Side=Right
  wires:
  Model/4 -> MX28 State/3
  Model/2 -> MX28 State/1
  Model/5 -> MX28 State/4
  Model/3 -> MX28 State/2
  Model/1 -> Torque converter/1
  MX28 Command/3 -> Model/5
  MX28 Command/6 -> Model/8
  MX28 Command/4 -> Model/6
  MX28 Command/5 -> Model/7
  MX28 Command/7 -> Model/9
  MX28 Command/2 -> Model/4
  MX28 Command/1 -> Model/3
  Position converter/1 -> Model/2
  Speed converter/1 -> Model/1
  Model/6 -> MX28 State/5
  MX28 Command/8 -> Model/10
  MX28 Command/9 -> Model/11
  connections:
  Axis/RConn1 -- Revolute Joint/RConn1 -- Inertia/RConn1
  Revolute Joint/LConn1 -- Base/RConn1
  Revolute Joint/RConn3 -- Speed converter/LConn1
  Revolute Joint/RConn2 -- Position converter/LConn1
  Revolute Joint/LConn2 -- Torque converter/RConn1

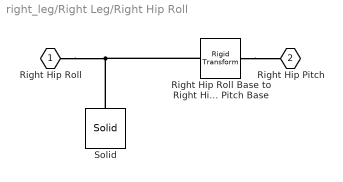
== system right_leg/Right Leg/Right Hip Roll ==
  Right Hip Roll Base to Right Hip Pitch Base : sm_lib/Frames and Transforms/Rigid Transform  TranslationMethod=Cartesian  TranslationLengthUnit=mm  TranslationStandardAxis=+Z  TranslationStandardOffset=0  TranslationCartesianOffset=[23.9 0 19.1]  TranslationROffset=0  TranslationROffsetUnits=m  TranslationZOffset=0  TranslationZOffsetUnits=m  TranslationThetaOffset=0  TranslationThetaOffsetUnits=deg  RotationMethod=AlignedAxes  RotationAngleUnits=deg  RotationStandardAxis=+Z  RotationAngle=0  RotationArbitraryAxis=[0 0 1]  FollAlignAxisA=+Z  BaseAlignAxisA=+X  FollAlignAxisB=+Y  BaseAlignAxisB=+Y  RotationMatrix=[1 0 0; 0 1 0; 0 0 1]  BlockFunction=simmechanics.library.frames_transforms.rigid_transform
  Solid : sm_lib/Body Elements/Solid  InertiaType=Custom  Mass=166.79  MassUnits=g  CenterOfMass=[-0.21 -11.21 1.04]  CenterOfMassUnits=mm  MomentsOfInertia=[11817 12213 6949]  MomentsOfInertiaUnits=g*mm^2  ProductsOfInertia=[4006 104 -199]  ProductsOfInertiaUnits=g*mm^2  DensityBased=on  Density=1000  DensityUnits=kg/(m^3)  GraphicType=FromGeometry  MarkerShape=Sphere  MarkerSize=10  MarkerSizeUnits=m  GraphicVisPropType=SimpleVisualProperties  GraphicDiffuseColor=[0.5 0.5 0.5]  GraphicSpecularColor=[0.5 0.5 0.5 1.0]  GraphicAmbientColor=[0.15 0.15 0.15 1.0]  GraphicEmissiveColor=[0.0 0.0 0.0 1.0]  GraphicShininess=75  GraphicOpacity=1.0  GeometryShape=FromFile  RectangleSize=[1 1]  RectangleSizeUnits=m  BrickDimensions=[1 1 1]  BrickDimensionUnits=mm  CylinderRadius=1  CylinderRadiusUnits=m  CylinderLength=1  CylinderLengthUnits=m  SphereRadius=1  SphereRadiusUnits=m  EllipsoidRadii=[1 1 1]  EllipsoidRadiiUnits=m  ExtrusionCrossSection=[1 1; -1 1; -1 -1; 1 -1]  ExtrusionCrossSectionUnits=m  ExtrusionLength=1  ExtrusionLengthUnits=m  PolygonNumSides=3  PolygonOuterRadius=1  PolygonOuterRadiusUnits=m  ExtGeomFileType=STL  ExtGeomFileName=D:\Ker Lann\systemes\darwin\kinematics\STL\Right_Hip2.STL  ExtGeomFileUnits=mm  RevolutionCrossSection=[1 1; 1 -1; 2 -1; 2 1]  RevolutionCrossSectionUnits=m  RevolutionExtent=Full  RevolutionAngle=180  RevolutionAngleUnits=deg  BlockFunction=simmechanics.library.body_elements.solid
  Right Hip Roll : PMIOPort  Port=1  Side=Left
  Right Hip Pitch : PMIOPort  Port=2  Side=Right
  connections:
  Right Hip Roll Base to Right Hip Pitch Base/LConn1 -- Solid/RConn1 -- Right Hip Roll/RConn1
  Right Hip Roll Base to Right Hip Pitch Base/RConn1 -- Right Hip Pitch/RConn1

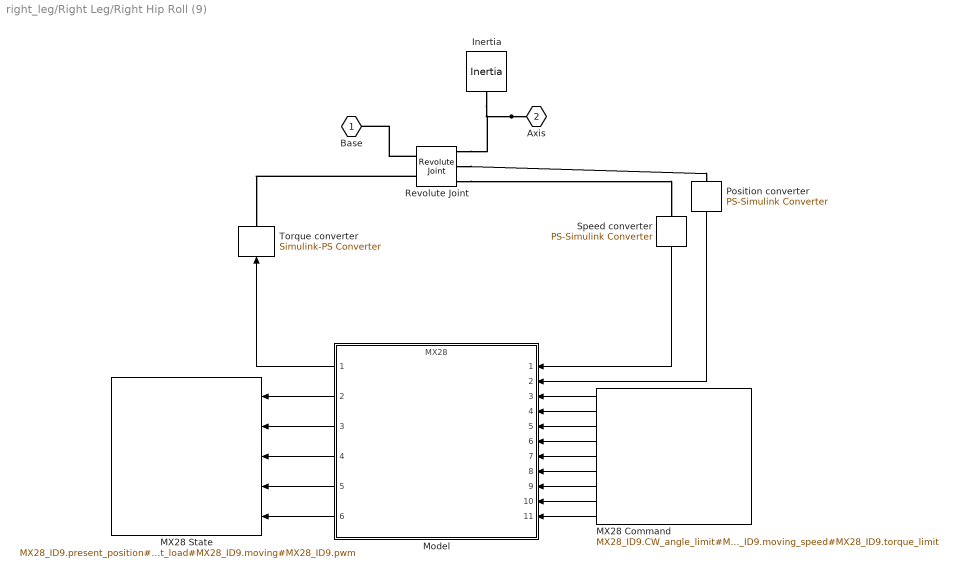
== system right_leg/Right Leg/Right Hip Roll (9) ==
  Inertia : sm_lib/Body Elements/Inertia  InertiaType=Custom  Mass=1  MassUnits=g  CenterOfMass=[0 0 0]  CenterOfMassUnits=m  MomentsOfInertia=[0 0 MX28_inertia]  MomentsOfInertiaUnits=kg*m^2  ProductsOfInertia=[0 0 0]  ProductsOfInertiaUnits=kg*m^2  BlockFunction=simmechanics.library.body_elements.inertia
  MX28 Command : DataStoreRead  DataStoreName=MX28_ID9  SampleTime=MX28_Te  DataStoreElements=MX28_ID9.CW_angle_limit#MX28_ID9.CCW_angle_limit#MX28_ID9.torque_enable#MX28_ID9.D_gain#MX28_ID9.I_gain#MX28_ID9.P_gain#MX28_ID9.goal_position#MX28_ID9.moving_speed#MX28_ID9.torque_limit
  MX28 State : DataStoreWrite  DataStoreName=MX28_ID9  DataStoreElements=MX28_ID9.present_position#MX28_ID9.present_speed#MX28_ID9.present_load#MX28_ID9.moving#MX28_ID9.pwm
  Model : ModelReference  ModelNameDialog=MX28.slx  SimulationMode=Normal  ModelReferenceVersion=1.66  CopyOfModelName=MX28.slx  DefaultDataLogging=on
  Position converter : nesl_utility/PS-Simulink Converter  PhysicalDomain=network_engine_domain  SubClassName=ps_output  LeftPortType=input  RightPortType=output  PseudoPeriodic=off  Frequencies=[]  Unit=rad  AffineConversion=off
  Revolute Joint : sm_lib/Joints/Revolute Joint  SenseConstraintForce=off  SenseConstraintForceX=off  SenseConstraintForceY=off  SenseConstraintForceZ=off  SenseConstraintTorque=off  SenseConstraintTorqueX=off  SenseConstraintTorqueY=off  SenseConstraintTorqueZ=off  SenseTotalForce=off  SenseTotalForceX=off  SenseTotalForceY=off  SenseTotalForceZ=off  SenseTotalTorque=off  SenseTotalTorqueX=off  SenseTotalTorqueY=off  SenseTotalTorqueZ=off  CompositeWrenchDir=FollowerOnBase  CompositeWrenchFrame=BaseFrame  EquilibriumPosition=0  EquilibriumPositionUnits=deg  SpringStiffness=0  SpringStiffnessUnits=N*m/deg  DampingCoefficient=MX28_lub_friction  DampingCoefficientUnits=N*m/(rad/s)  TorqueActuationMode=InputTorque  MotionActuationMode=ComputedMotion  SensePosition=on  SenseVelocity=on  SenseAcceleration=off  SenseTorqueForce=off  PositionTargetValue=MX28_init_position  PositionTargetValueUnits=rad  PositionTargetSpecify=on  PositionTargetPriority=High  VelocityTargetValue=MX28_init_speed  VelocityTargetValueUnits=rad/s  VelocityTargetSpecify=on  VelocityTargetPriority=High  BlockFunction=simmechanics.library.joints.revolute_joint
  Speed converter : nesl_utility/PS-Simulink Converter  PhysicalDomain=network_engine_domain  SubClassName=ps_output  LeftPortType=input  RightPortType=output  PseudoPeriodic=off  Frequencies=[]  Unit=rad/s  AffineConversion=off
  Torque converter : nesl_utility/Simulink-PS Converter  PhysicalDomain=network_engine_domain  SubClassName=ps_input  LeftPortType=input  RightPortType=output  PseudoPeriodic=off  Frequencies=[]  NoiseDistribution=none  NoiseParameters=[]  Unit=N*m  AffineConversion=off  InputFiltering=off  SimscapeFilterOrder=1  InputFilterTimeConstant=0.001  UdotUserProvided=1
  Base : PMIOPort  Port=1  Side=Left
  Axis : PMIOPort  Port=2  Side=Right
  wires:
  Model/4 -> MX28 State/3
  Model/2 -> MX28 State/1
  Model/5 -> MX28 State/4
  Model/3 -> MX28 State/2
  Model/1 -> Torque converter/1
  MX28 Command/3 -> Model/5
  MX28 Command/6 -> Model/8
  MX28 Command/4 -> Model/6
  MX28 Command/5 -> Model/7
  MX28 Command/7 -> Model/9
  MX28 Command/2 -> Model/4
  MX28 Command/1 -> Model/3
  Position converter/1 -> Model/2
  Speed converter/1 -> Model/1
  Model/6 -> MX28 State/5
  MX28 Command/8 -> Model/10
  MX28 Command/9 -> Model/11
  connections:
  Axis/RConn1 -- Revolute Joint/RConn1 -- Inertia/RConn1
  Revolute Joint/LConn1 -- Base/RConn1
  Revolute Joint/RConn3 -- Speed converter/LConn1
  Revolute Joint/RConn2 -- Position converter/LConn1
  Revolute Joint/LConn2 -- Torque converter/RConn1

== system right_leg/Right Leg/Right Hip Yaw ==
  Right Hip Yaw Axis to Right Hip Roll Axis : sm_lib/Frames and Transforms/Rigid Transform  TranslationMethod=Cartesian  TranslationLengthUnit=mm  TranslationStandardAxis=+Z  TranslationStandardOffset=0  TranslationCartesianOffset=[24.85 0 28.35]  TranslationROffset=0  TranslationROffsetUnits=m  TranslationZOffset=0  TranslationZOffsetUnits=m  TranslationThetaOffset=0  TranslationThetaOffsetUnits=deg  RotationMethod=AlignedAxes  RotationAngleUnits=deg  RotationStandardAxis=+Z  RotationAngle=0  RotationArbitraryAxis=[0 0 1]  FollAlignAxisA=+Y  BaseAlignAxisA=+Z  FollAlignAxisB=+X  BaseAlignAxisB=-Y  RotationMatrix=[1 0 0; 0 1 0; 0 0 1]  BlockFunction=simmechanics.library.frames_transforms.rigid_transform
  Solid : sm_lib/Body Elements/Solid  InertiaType=Custom  Mass=34.1  MassUnits=g  CenterOfMass=[7.53 0 10.27]  CenterOfMassUnits=mm  MomentsOfInertia=[8263 18980 13482]  MomentsOfInertiaUnits=g*mm^2  ProductsOfInertia=[0 3667 0]  ProductsOfInertiaUnits=g*mm^2  DensityBased=on  Density=1000  DensityUnits=kg/(m^3)  GraphicType=FromGeometry  MarkerShape=Sphere  MarkerSize=10  MarkerSizeUnits=m  GraphicVisPropType=SimpleVisualProperties  GraphicDiffuseColor=[0.5 0.5 0.5]  GraphicSpecularColor=[0.5 0.5 0.5 1.0]  GraphicAmbientColor=[0.15 0.15 0.15 1.0]  GraphicEmissiveColor=[0.0 0.0 0.0 1.0]  GraphicShininess=75  GraphicOpacity=1.0  GeometryShape=FromFile  RectangleSize=[1 1]  RectangleSizeUnits=m  BrickDimensions=[1 1 1]  BrickDimensionUnits=mm  CylinderRadius=1  CylinderRadiusUnits=m  CylinderLength=1  CylinderLengthUnits=m  SphereRadius=1  SphereRadiusUnits=m  EllipsoidRadii=[1 1 1]  EllipsoidRadiiUnits=m  ExtrusionCrossSection=[1 1; -1 1; -1 -1; 1 -1]  ExtrusionCrossSectionUnits=m  ExtrusionLength=1  ExtrusionLengthUnits=m  PolygonNumSides=3  PolygonOuterRadius=1  PolygonOuterRadiusUnits=m  ExtGeomFileType=STL  ExtGeomFileName=D:\Ker Lann\systemes\darwin\kinematics\STL\Hip1.STL  ExtGeomFileUnits=mm  RevolutionCrossSection=[1 1; 1 -1; 2 -1; 2 1]  RevolutionCrossSectionUnits=m  RevolutionExtent=Full  RevolutionAngle=180  RevolutionAngleUnits=deg  BlockFunction=simmechanics.library.body_elements.solid
  Right Hip Yaw : PMIOPort  Port=1  Side=Left
  Right Hip Roll : PMIOPort  Port=2  Side=Right
  connections:
  Right Hip Yaw Axis to Right Hip Roll Axis/RConn1 -- Right Hip Roll/RConn1
  Solid/RConn1 -- Right Hip Yaw Axis to Right Hip Roll Axis/LConn1 -- Right Hip Yaw/RConn1

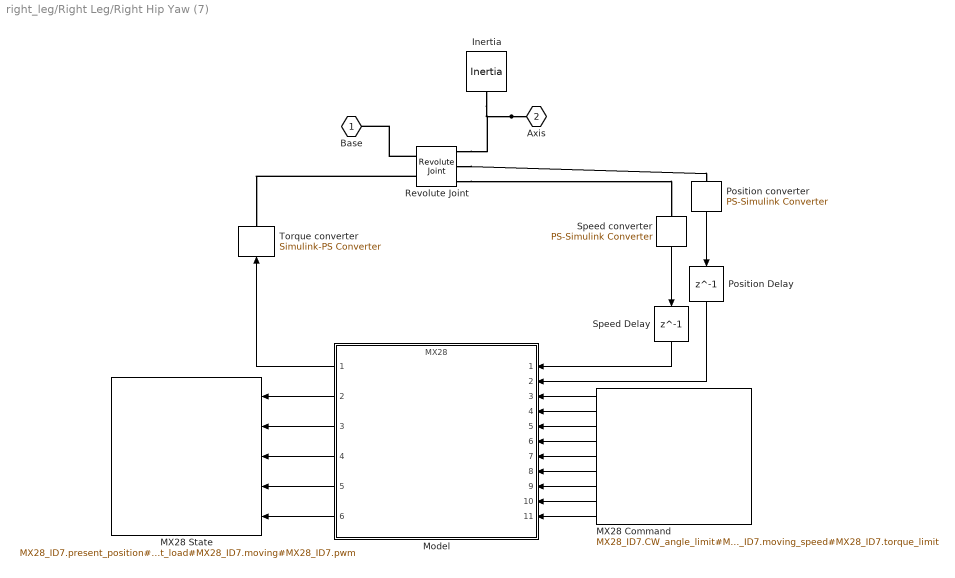
== system right_leg/Right Leg/Right Hip Yaw (7) ==
  Inertia : sm_lib/Body Elements/Inertia  InertiaType=Custom  Mass=1  MassUnits=g  CenterOfMass=[0 0 0]  CenterOfMassUnits=m  MomentsOfInertia=[0 0 MX28_inertia]  MomentsOfInertiaUnits=kg*m^2  ProductsOfInertia=[0 0 0]  ProductsOfInertiaUnits=kg*m^2  BlockFunction=simmechanics.library.body_elements.inertia
  MX28 Command : DataStoreRead  DataStoreName=MX28_ID7  SampleTime=MX28_Te  DataStoreElements=MX28_ID7.CW_angle_limit#MX28_ID7.CCW_angle_limit#MX28_ID7.torque_enable#MX28_ID7.D_gain#MX28_ID7.I_gain#MX28_ID7.P_gain#MX28_ID7.goal_position#MX28_ID7.moving_speed#MX28_ID7.torque_limit
  MX28 State : DataStoreWrite  DataStoreName=MX28_ID7  DataStoreElements=MX28_ID7.present_position#MX28_ID7.present_speed#MX28_ID7.present_load#MX28_ID7.moving#MX28_ID7.pwm
  Model : ModelReference  ModelNameDialog=MX28.slx  SimulationMode=Normal  ModelReferenceVersion=1.66  CopyOfModelName=MX28.slx  DefaultDataLogging=on
  Position Delay : Delay  DelayLength=1  InitialCondition=MX28_init_position  SampleTime=MX28_Te
  Position converter : nesl_utility/PS-Simulink Converter  PhysicalDomain=network_engine_domain  SubClassName=ps_output  LeftPortType=input  RightPortType=output  PseudoPeriodic=off  Frequencies=[]  Unit=rad  AffineConversion=off
  Revolute Joint : sm_lib/Joints/Revolute Joint  SenseConstraintForce=off  SenseConstraintForceX=off  SenseConstraintForceY=off  SenseConstraintForceZ=off  SenseConstraintTorque=off  SenseConstraintTorqueX=off  SenseConstraintTorqueY=off  SenseConstraintTorqueZ=off  SenseTotalForce=off  SenseTotalForceX=off  SenseTotalForceY=off  SenseTotalForceZ=off  SenseTotalTorque=off  SenseTotalTorqueX=off  SenseTotalTorqueY=off  SenseTotalTorqueZ=off  CompositeWrenchDir=FollowerOnBase  CompositeWrenchFrame=BaseFrame  EquilibriumPosition=0  EquilibriumPositionUnits=deg  SpringStiffness=0  SpringStiffnessUnits=N*m/deg  DampingCoefficient=MX28_lub_friction  DampingCoefficientUnits=N*m/(rad/s)  TorqueActuationMode=InputTorque  MotionActuationMode=ComputedMotion  SensePosition=on  SenseVelocity=on  SenseAcceleration=off  SenseTorqueForce=off  PositionTargetValue=MX28_init_position  PositionTargetValueUnits=rad  PositionTargetSpecify=on  PositionTargetPriority=High  VelocityTargetValue=MX28_init_speed  VelocityTargetValueUnits=rad/s  VelocityTargetSpecify=on  VelocityTargetPriority=High  BlockFunction=simmechanics.library.joints.revolute_joint
  Speed Delay : Delay  DelayLength=1  InitialCondition=MX28_init_speed  SampleTime=MX28_Te
  Speed converter : nesl_utility/PS-Simulink Converter  PhysicalDomain=network_engine_domain  SubClassName=ps_output  LeftPortType=input  RightPortType=output  PseudoPeriodic=off  Frequencies=[]  Unit=rad/s  AffineConversion=off
  Torque converter : nesl_utility/Simulink-PS Converter  PhysicalDomain=network_engine_domain  SubClassName=ps_input  LeftPortType=input  RightPortType=output  PseudoPeriodic=off  Frequencies=[]  NoiseDistribution=none  NoiseParameters=[]  Unit=N*m  AffineConversion=off  InputFiltering=off  SimscapeFilterOrder=1  InputFilterTimeConstant=0.001  UdotUserProvided=1
  Base : PMIOPort  Port=1  Side=Left
  Axis : PMIOPort  Port=2  Side=Right
  wires:
  Model/4 -> MX28 State/3
  Model/2 -> MX28 State/1
  Model/5 -> MX28 State/4
  Model/3 -> MX28 State/2
  Model/1 -> Torque converter/1
  Speed converter/1 -> Speed Delay/1
  Position converter/1 -> Position Delay/1
  MX28 Command/3 -> Model/5
  MX28 Command/6 -> Model/8
  MX28 Command/4 -> Model/6
  MX28 Command/5 -> Model/7
  MX28 Command/7 -> Model/9
  MX28 Command/2 -> Model/4
  MX28 Command/1 -> Model/3
  Position Delay/1 -> Model/2
  Speed Delay/1 -> Model/1
  Model/6 -> MX28 State/5
  MX28 Command/8 -> Model/10
  MX28 Command/9 -> Model/11
  connections:
  Axis/RConn1 -- Revolute Joint/RConn1 -- Inertia/RConn1
  Revolute Joint/LConn1 -- Base/RConn1
  Revolute Joint/RConn3 -- Speed converter/LConn1
  Revolute Joint/RConn2 -- Position converter/LConn1
  Revolute Joint/LConn2 -- Torque converter/RConn1
